simulink model "I_OShard_OSsoft_x1"  (Simulink 5.0)
settings: Solver=ode45  StartTime=0.0  StopTime=20  RelTol=1e-3
settings Model: LastModifiedBy=User  BlockReductionOpt=off  BooleanDataType=off

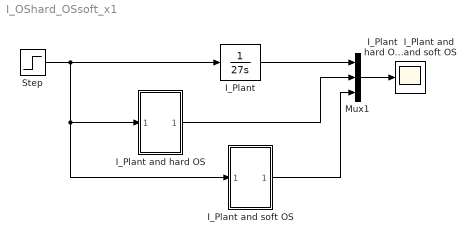
== system I_OShard_OSsoft_x1 ==
  I_Plant : TransferFcn  Denominator=[27 0]
  I_Plant  I_Plant and hard OS I_Plant and soft OS : Scope
      settings: YMin=-5e+283  YMax=9e+284
  I_Plant and hard OS : Subsystem
  I_Plant and soft OS : Subsystem
  Mux1 : Mux  Inputs=3
  Step : Step  Time=0.1  SampleTime=0
  wires:
  Step/1 -> I_Plant/1, I_Plant and hard OS/1(In1), I_Plant and soft OS/1(In1)
  I_Plant/1 -> Mux1/1
  Mux1/1 -> I_Plant  I_Plant and hard OS I_Plant and soft OS/1
  I_Plant and hard OS/1(Out1) -> Mux1/2
  I_Plant and soft OS/1(Out1) -> Mux1/3

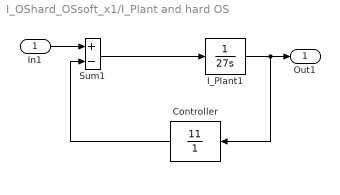
== system I_OShard_OSsoft_x1/I_Plant and hard OS ==
  In1 : Inport
  Controller : TransferFcn  Orientation=left  Numerator=[11]  Denominator=[0 1]
  I_Plant1 : TransferFcn  Denominator=[27 0]
  Sum1 : Sum  Inputs=+-  SaturateOnIntegerOverflow=on  InputSameDT=on
  Out1 : Outport
  wires:
  Sum1/1 -> I_Plant1/1
  I_Plant1/1 -> Controller/1, Out1/1
  Controller/1 -> Sum1/2
  In1/1 -> Sum1/1

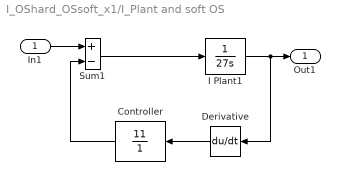
== system I_OShard_OSsoft_x1/I_Plant and soft OS ==
  In1 : Inport
  Controller : TransferFcn  Orientation=left  Numerator=[11]  Denominator=[0 1]
  Derivative : Derivative  Orientation=left
  I Plant1 : TransferFcn  Denominator=[27 0]
  Sum1 : Sum  Inputs=+-  SaturateOnIntegerOverflow=on  InputSameDT=on
  Out1 : Outport
  wires:
  Sum1/1 -> I Plant1/1
  I Plant1/1 -> Derivative/1, Out1/1
  Controller/1 -> Sum1/2
  Derivative/1 -> Controller/1
  In1/1 -> Sum1/1
